simulink model "series_form_2nd"  (R2023b)
settings: Solver=VariableStepAuto  StartTime=0.0  StopTime=10.0  RelTol=1e-3
undefined symbols (not defined in the file): a1, a2, b1, b2
settings Model: Creator=eechris  LastModifiedBy=eechris

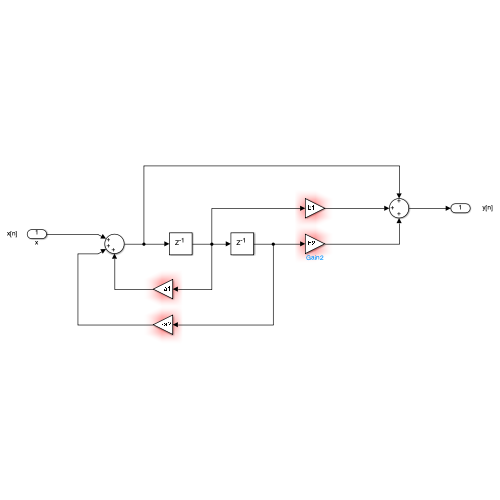
[thumbnail: Simulink's stored preview of the top-level diagram]
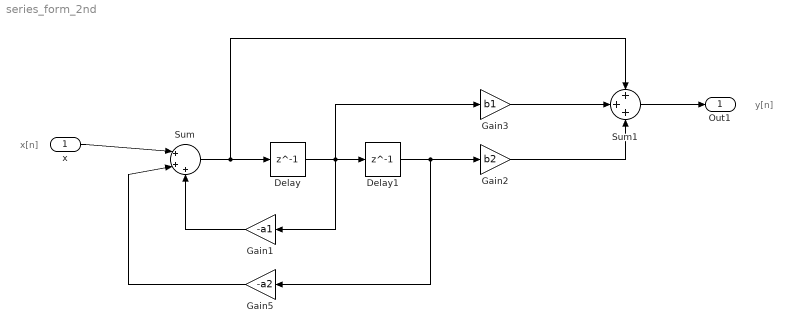
== system series_form_2nd ==
  note: x[n]
  note: y[n]
  x : Inport
  Delay : Delay  DelayLength=1  InitialCondition=0
  Delay1 : Delay  DelayLength=1  InitialCondition=0
  Gain1 : Gain  Gain=-a1
  Gain2 : Gain  Gain=b2
  Gain3 : Gain  Gain=b1
  Gain5 : Gain  Gain=-a2
  Sum : Sum  Inputs=|+++
  Sum1 : Sum  Inputs=+++
  Out1 : Outport
  wires:
  Delay/1 -> Gain1/1, Gain3/1, Delay1/1
  Delay1/1 -> Gain5/1, Gain2/1
  Sum/1 -> Sum1/1, Delay/1
  x/1 -> Sum/1
  Gain3/1 -> Sum1/2
  Gain2/1 -> Sum1/3
  Sum1/1 -> Out1/1
  Gain5/1 -> Sum/2
  Gain1/1 -> Sum/3
